simulink model "Chaine_de_conversion_eolienne_25kw"  (R2024a)
settings: Solver=FixedStepAuto  StartTime=0.0  StopTime=10  FixedStep=Ts  RelTol=1e-3
undefined symbols (not defined in the file): A1, A2, A3, A4, A5, A6, C_dc, f, F, G, J, J_PMSG, ki_id_grid, ki_iq_grid, ki_isd, ki_omega, ki_PLL, ki_Q, ki_vdc, kp_id_grid, kp_iq_grid, kp_isd, kp_omega, kp_PLL, kp_Q, kp_vdc, Kt, Lf, Ls, p, Phi_r, R, Rf, rho, Rs, S, Ts, Vdc_ref
libraries: eeGeneralControl x12, slpidlib x8, spsThreePhaseVIMeasurementLib x3, eeTransforms x3, spsCurrentMeasurementLib x3, spsVoltageMeasurementLib x3, spsUniversalBridgeLib x2, spsPWMGenerator2LevelLib x2, powerlib_extras x2, spsRMSLib x2, spsTHDLib x2, spsThreePhaseSeriesRLCBranchLib x1
(part 1 of 2)
settings Model: Creator=K Edd Edd  LastModifiedBy=K Edd Edd
settings DataIOCC: SignalLogging=off  DSMLogging=off  ReturnWorkspaceOutputs=off

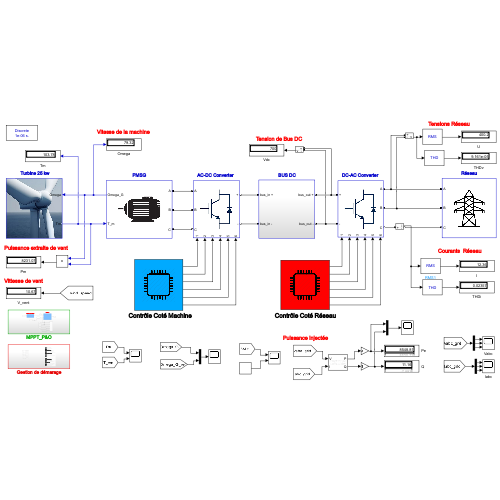
[thumbnail: Simulink's stored preview of the top-level diagram]
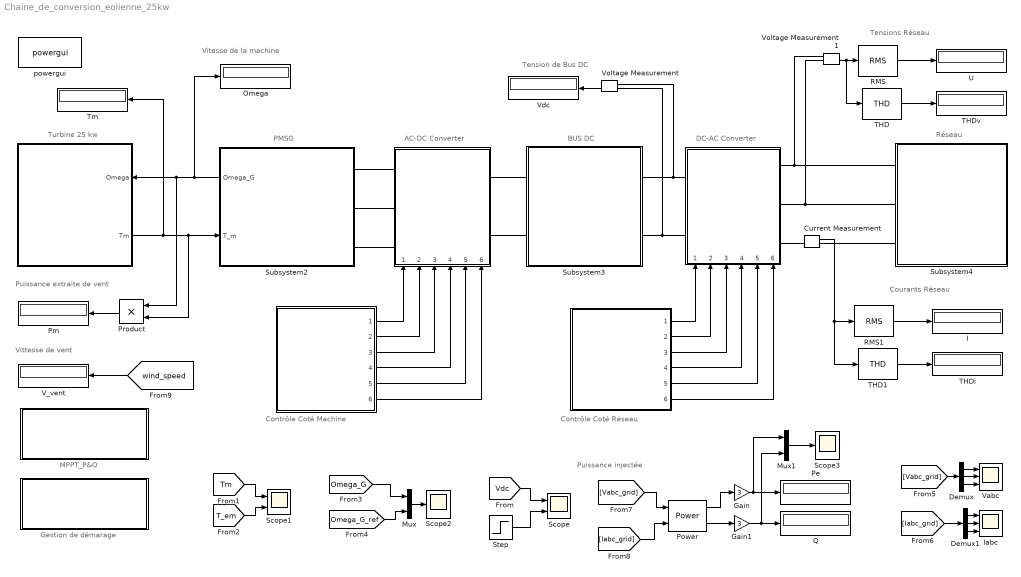
== system Chaine_de_conversion_eolienne_25kw ==
  note: Courants Réseau
  note: MPPT_P&O
  note: Turbine 25 kw
  note: PMSG
  note: AC-DC Converter
  note: BUS DC
  note: DC-AC Converter
  note: Réseau
  note: Gestion de démarage
  note: Contrôle Coté Machine
  note: Tensions Réseau
  note: Puissance injectée
  note: Tension de Bus DC
  note: Vitesse de la machine
  note: Puissance extraite de vent
  note: Contrôle Coté Réseau
  note: Vittesse de vent
  "  " : Subsystem
      settings: PortSchema="{\"entries\":[{\"content\":{\"sides\":[{\"content\":{\"connectorIds\":[\"LConn1\",\"LConn2\",\"LConn3\"]},\"type\":\"ConnectorPlacement.EquallySpacedRectSide\",\"uuid\":\"aa5a1e19-58e8-4f63-9a1b-77e9bc10e920\"},{\"content\":{\"connectorIds\":[\"RConn1\",\"RConn2\"],\"side\":\"RIGHT\"},\"type\":\"ConnectorPlacement.EquallySpacedRectSide\",\"uuid\":\"2d85d2be-ece1-4429-a3f7-d4ed68196552\"},{\"content\":{\"side\":\"TOP\"},\"type\":\"ConnectorPlacement.EquallySpacedRectSide\",\"uuid\":\"982ebd7b-1595-4ee8-b406-473be6344857\"},{\"content\":{\"connectorIds\":[\"In1\",\"In2\",\"In3\",\"In4\",\"In5\",\"In6\"],\"side\":\"BOTTOM\"},\"type\":\"ConnectorPlacement.EquallySpacedRectSide\",\"uuid\":\"f79fcda1-556e-4eeb-b27d-f3a2253a7ec4\"}]},\"type\":\"ConnectorPlacement.EquallySpacedConnector\",\"uuid\":\"743085b1-d620-4124-a445-722ff99a9231\"}],\"packageUris\":[\"http://schema.mathworks.com/mf0/Connector/R2020b\"],\"version\":\"1.0\"}"
      mask Display: image('Bridge_3ph.png', [0,0,0,0,90,90]);
  "   " : Subsystem
      settings: PortSchema="{\"entries\":[{\"content\":{\"sides\":[{\"content\":{},\"type\":\"ConnectorPlacement.EquallySpacedRectSide\",\"uuid\":\"46343f75-74e6-4f4c-9efc-4b43e6213925\"},{\"content\":{\"connectorIds\":[\"In1\",\"Out1\"],\"side\":\"RIGHT\"},\"type\":\"ConnectorPlacement.EquallySpacedRectSide\",\"uuid\":\"10880a8c-ba30-44f8-b93e-97455e8769b4\"},{\"content\":{\"side\":\"TOP\"},\"type\":\"ConnectorPlacement.EquallySpacedRectSide\",\"uuid\":\"fc9f6e01-6aae-438b-b3e4-23506a1fb9e3\"}]},\"type\":\"ConnectorPlacement.EquallySpacedConnector\",\"uuid\":\"29e446f6-be91-4db2-b818-9d2408c26281\"}],\"packageUris\":[\"http://schema.mathworks.com/mf0/Connector/R2020b\"],\"version\":\"1.0\"}"
      mask Display: image('Turbine.jpg');
  "    " : Subsystem
  "      " : Subsystem
  "         " : Subsystem
      settings: PortSchema="{\"entries\":[{\"content\":{\"sides\":[{\"content\":{\"connectorIds\":[\"LConn1\",\"LConn2\"]},\"type\":\"ConnectorPlacement.EquallySpacedRectSide\",\"uuid\":\"6a59fa23-55cb-493a-902b-27daa7c75780\"},{\"content\":{\"connectorIds\":[\"RConn1\",\"RConn2\",\"RConn3\"],\"side\":\"RIGHT\"},\"type\":\"ConnectorPlacement.EquallySpacedRectSide\",\"uuid\":\"f4ee7100-af9b-4531-bfab-eaffe06050e9\"},{\"content\":{\"side\":\"TOP\"},\"type\":\"ConnectorPlacement.EquallySpacedRectSide\",\"uuid\":\"b4ec731b-d05c-4ff1-948d-ff2fdeb075f1\"},{\"content\":{\"connectorIds\":[\"In1\",\"In2\",\"In3\",\"In4\",\"In5\",\"In6\"],\"side\":\"BOTTOM\"},\"type\":\"ConnectorPlacement.EquallySpacedRectSide\",\"uuid\":\"1fd09039-83e1-473e-9ccb-1d87c041e7c6\"}]},\"type\":\"ConnectorPlacement.EquallySpacedConnector\",\"uuid\":\"54ae46ec-08f8-45c2-a8da-c49a7efba60c\"}],\"packageUris\":[\"http://schema.mathworks.com/mf0/Connector/R2020b\"],\"version\":\"1.0\"}"
      mask Display: image('Bridge_3ph.png', [0,0,0,0,90,90]);
  "                 " : Subsystem
      settings: PortSchema="{\"entries\":[{\"content\":{\"sides\":[{\"content\":{},\"type\":\"ConnectorPlacement.EquallySpacedRectSide\",\"uuid\":\"68bdff09-e8ec-4d6d-b05e-55201ee357f5\"},{\"content\":{\"side\":\"RIGHT\"},\"type\":\"ConnectorPlacement.EquallySpacedRectSide\",\"uuid\":\"a14a2bca-9db8-408e-b5bf-8e3869a2fb13\"},{\"content\":{\"connectorIds\":[\"Out1\",\"Out2\",\"Out3\",\"Out4\",\"Out5\",\"Out6\"],\"side\":\"TOP\"},\"type\":\"ConnectorPlacement.EquallySpacedRectSide\",\"uuid\":\"600d12f1-b4e8-4864-955c-a539efb19c99\"}]},\"type\":\"ConnectorPlacement.EquallySpacedConnector\",\"uuid\":\"05b2b3d9-6bdc-4d72-9457-a6c68afa543f\"}],\"packageUris\":[\"http://schema.mathworks.com/mf0/Connector/R2020b\"],\"version\":\"1.0\"}"
      mask Display: image('Cotroller.jpg', [0,0,0,0,70,70]);
  "                       " : Subsystem
      settings: PortSchema="{\"entries\":[{\"content\":{\"sides\":[{\"content\":{},\"type\":\"ConnectorPlacement.EquallySpacedRectSide\",\"uuid\":\"68bdff09-e8ec-4d6d-b05e-55201ee357f5\"},{\"content\":{\"side\":\"RIGHT\"},\"type\":\"ConnectorPlacement.EquallySpacedRectSide\",\"uuid\":\"a14a2bca-9db8-408e-b5bf-8e3869a2fb13\"},{\"content\":{\"connectorIds\":[\"Out1\",\"Out2\",\"Out3\",\"Out4\",\"Out5\",\"Out6\"],\"side\":\"TOP\"},\"type\":\"ConnectorPlacement.EquallySpacedRectSide\",\"uuid\":\"600d12f1-b4e8-4864-955c-a539efb19c99\"}]},\"type\":\"ConnectorPlacement.EquallySpacedConnector\",\"uuid\":\"05b2b3d9-6bdc-4d72-9457-a6c68afa543f\"}],\"packageUris\":[\"http://schema.mathworks.com/mf0/Connector/R2020b\"],\"version\":\"1.0\"}"
      mask Display: image('Cotroller.jpg', [0,0,0,0,70,70]);
  Current Measurement : spsCurrentMeasurementLib/Current Measurement  PhasorSimulation=off  OutputType=Complex  PSBequivalent=0
  Demux : Demux  Outputs=3
  Demux1 : Demux  Outputs=3
  Gain : Gain  Gain=3
  Gain1 : Gain  Gain=3
  I : Display
  Iabc : Scope  NumInputPorts=3
  Mux : Mux  Inputs=2
  Mux1 : Mux  Inputs=2
  Omega : Display
  Pe : Display
      settings: Format=bank
  Pm : Display
      settings: Format=bank
  Power : spsPowerLib/Power  Freq=50  Vinit=[0, 0]  Iinit=[0, 0]  Ts=0
  Product : Product
  Q : Display
  RMS : spsRMSLib/RMS  TrueRMS=on  Freq=50  RMSInit=0  Ts=Ts
  RMS1 : spsRMSLib/RMS  TrueRMS=on  Freq=50  RMSInit=0  Ts=Ts
  Scope : Scope  NumInputPorts=2
  Scope1 : Scope  NumInputPorts=2
  Scope2 : Scope
  Scope3 : Scope
  Step : Step  Time=1e-8  Before=1e-8  After=700  SampleTime=0
  Subsystem2 : Subsystem
      settings: PortSchema="{\"entries\":[{\"content\":{\"sides\":[{\"content\":{\"connectorIds\":[\"Out1\",\"In1\"]},\"type\":\"ConnectorPlacement.EquallySpacedRectSide\",\"uuid\":\"3f25ae88-b85d-4aa8-83e0-c8881128a15f\"},{\"content\":{\"connectorIds\":[\"RConn1\",\"RConn2\",\"RConn3\"],\"side\":\"RIGHT\"},\"type\":\"ConnectorPlacement.EquallySpacedRectSide\",\"uuid\":\"21769176-b893-4bdb-b404-3c9a8a9ec7d7\"},{\"content\":{\"side\":\"TOP\"},\"type\":\"ConnectorPlacement.EquallySpacedRectSide\",\"uuid\":\"6b86daf7-1109-4b9d-a4e1-050e61d06be5\"}]},\"type\":\"ConnectorPlacement.EquallySpacedConnector\",\"uuid\":\"4237b530-1620-4b33-bc88-1364db079d0f\"}],\"packageUris\":[\"http://schema.mathworks.com/mf0/Connector/R2020b\"],\"version\":\"1.0\"}"
      mask Display: image('Machine.jpg');
  Subsystem3 : Subsystem
  Subsystem4 : Subsystem
      mask Display: image('Grid.jpg', [0,0,0,0,80,80]);
  THD : spsTHDLib/THD  Freq=50  Ts=0
  THD1 : spsTHDLib/THD  Freq=50  Ts=0
  THDi : Display
  THDv : Display
  Tm : Display
      settings: Format=bank
  U : Display
  V_vent : Display
      settings: Format=bank
  Vabc : Scope  NumInputPorts=3
  Vdc : Display
  Voltage Measurement : spsVoltageMeasurementLib/Voltage Measurement  PhasorSimulation=off  OutputType=Complex  PSBequivalent=0
  Voltage Measurement1 : spsVoltageMeasurementLib/Voltage Measurement  PhasorSimulation=off  OutputType=Complex  PSBequivalent=0
  powergui : sps_lib/powergui  Priority=1  SimulationMode=Discrete  SampleTime=Ts  frequency=60  Iterations=50  frequencyindice=0  Pbase=100e6  ErrMax=1e-4  UnitsV=kV  UnitsW=MW  buscounter=0  FunctionMessages=off  echomessages=off  EnableUseOfTLC=off  CurrentSourceSwitches=off  DisableSnubberDevices=off  DisableRonSwitches=off  DisableVfSwitches=off  DisplayEquations=off  AutomaticDiscreteSolvers=off  SolverType=Tustin/Backward Euler (TBE)  Interpol=off  ExternalGateDelay=off  methode=off  Ts=100  x0status=blocks  SPID=on  SwTol=0  HookPort=off  NonlinearTolerance=1e-4  nMaxIteration=100  ContinueOnMaxIteration=off  RestoreLinks=warning  ResistiveCurrentMeasurement=off  Frange=[0:2:500]  Ylog=off  Xlog=on  ShowGrid=off  save=off  variable=ZData  structure=0  ZoomFFT=off  StartTime=0.0  cycles=1  DisplayStyle=1  fundamental=60  FreqAxis=off  MaxFrequency=1000  frequencyindicesteady=1  RmsSteady=1  display=off
  wires:
  "                 "/1(" ") -> "  "/1(Input)
  "                 "/2("  ") -> "  "/2(Input1)
  "                 "/3("   ") -> "  "/3(Input2)
  "                 "/4("    ") -> "  "/4(Input3)
  "                 "/5("     ") -> "  "/5(Input4)
  "                 "/6("       ") -> "  "/6(Input5)
  "   "/1(Tm) -> Tm/1, Product/2, Subsystem2/1(T_m)
  "                       "/4("    ") -> "         "/4(Input3)
  "                       "/6("      ") -> "         "/6(Input5)
  "                       "/3("   ") -> "         "/3(Input2)
  "                       "/1(" ") -> "         "/1(Input)
  "                       "/2("  ") -> "         "/2(Input1)
  "                       "/5("     ") -> "         "/5(Input4)
  Voltage Measurement/1 -> Vdc/1
  Voltage Measurement1/1 -> RMS/1, THD/1
  RMS/1 -> U/1
  THD/1 -> THDv/1
  Demux1/3 -> Iabc/3
  Demux/1 -> Vabc/1
  [Iabc_grid] -> Demux1/1
  Demux1/2 -> Iabc/2
  Demux/3 -> Vabc/3
  Demux1/1 -> Iabc/1
  Demux/2 -> Vabc/2
  [Vabc_grid] -> Demux/1
  [Vdc] -> Scope/1
  Step/1 -> Scope/2
  [T_em] -> Scope1/2
  [Tm] -> Scope1/1
  Product/1 -> Pm/1
  Subsystem2/1(Omega_G) -> "   "/1(Omega), Product/1, Omega/1
  [Vabc_grid] -> Power/1
  [Iabc_grid] -> Power/2
  Power/1 -> Gain/1
  Power/2 -> Gain1/1
  Gain1/1 -> Mux1/2, Q/1
  THD1/1 -> THDi/1
  RMS1/1 -> I/1
  Current Measurement/1 -> RMS1/1, THD1/1
  [wind_speed] -> V_vent/1
  [Omega_G] -> Mux/1
  Mux/1 -> Scope2/1
  [Omega_G_ref] -> Mux/2
  Mux1/1 -> Scope3/1
  Gain/1 -> Mux1/1, Pe/1
  connections:
  Subsystem2/RConn1 -- "  "/LConn1
  Subsystem2/RConn2 -- "  "/LConn2
  Subsystem2/RConn3 -- "  "/LConn3
  Subsystem3/LConn1 -- "  "/RConn1
  "  "/RConn2 -- Subsystem3/LConn2
  "         "/LConn1 -- Voltage Measurement/LConn1 -- Subsystem3/RConn1
  "         "/LConn2 -- Voltage Measurement/LConn2 -- Subsystem3/RConn2
  Subsystem4/LConn1 -- Voltage Measurement1/LConn1 -- "         "/RConn1
  Subsystem4/LConn2 -- Voltage Measurement1/LConn2 -- "         "/RConn2
  Current Measurement/LConn1 -- "         "/RConn3
  Current Measurement/RConn1 -- Subsystem4/LConn3

== system Chaine_de_conversion_eolienne_25kw/   ==
  note: Redresseur actif
  note: Bus DC
  note: Tensions Machine
  Input : Inport
  Input1 : Inport  Port=2
  Input2 : Inport  Port=3
  Input3 : Inport  Port=4
  Input4 : Inport  Port=5
  Input5 : Inport  Port=6
  "  " : spsUniversalBridgeLib/Universal Bridge  Arms=3  SnubberResistance=1e7  SnubberCapacitance=inf  Device=IGBT / Diodes  Ron=1e-2  Lon=0  ForwardVoltages="[  0  0  ]"  ForwardVoltage=0  GTOparameters=[ 10e-6 , 20e-6 ]  IGBTparameters=[ 0 , 0 ]  Measurements=None  Measurements_2=None  converterType=Rectifier
  Mux : Mux  Inputs=6
  A : PMIOPort  Side=Left
  B : PMIOPort  Port=2  Side=Left
  C : PMIOPort  Port=3  Side=Left
  + : PMIOPort  Port=4  Side=Right
  - : PMIOPort  Port=5  Side=Right
  wires:
  Input/1 -> Mux/1
  Input1/1 -> Mux/2
  Input2/1 -> Mux/3
  Input3/1 -> Mux/4
  Input4/1 -> Mux/5
  Input5/1 -> Mux/6
  Mux/1 -> "  "/1
  connections:
  -/RConn1 -- "  "/RConn2
  B/RConn1 -- "  "/LConn2
  A/RConn1 -- "  "/LConn1
  C/RConn1 -- "  "/LConn3
  +/RConn1 -- "  "/RConn1

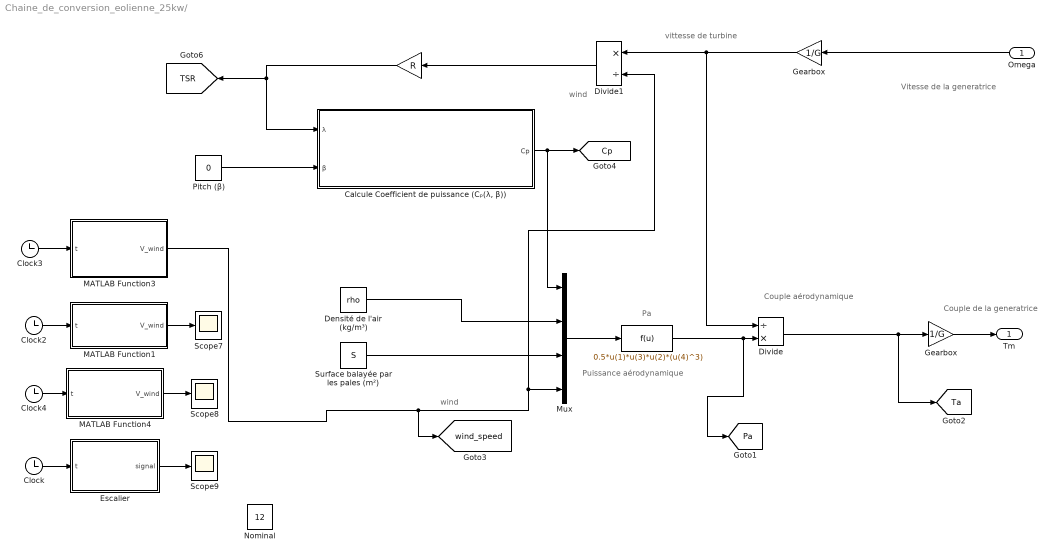
== system Chaine_de_conversion_eolienne_25kw/    ==
  note: Couple de la generatrice
  note: Puissance aérodynamique
  note: wind
  note: vittesse de turbine
  note: Couple aérodynamique
  note: Vitesse de la generatrice
  note: Pa
  note: wind
  Omega : Inport
  "  " : Fcn  Expr=0.5*u(1)*u(3)*u(2)*(u(4)^3)
  "   " : Gain  Gain=R
  "Calcule Coefficient de puissance (Cₚ(λ, β))" : Subsystem
  Clock{,2..4} (4 alike) : Clock
  Densité de l'air (kg/m³) : Constant  Value=rho
  Divide : Product  Inputs=/*
  Divide1 : Product  Inputs=*/
  Escalier : MATLAB Function  TreatAsAtomicUnit=on
  Gearbox : Gain  Gain=1/G
  "Gearbox   " : Gain  Gain=1/G
  MATLAB Function1 : MATLAB Function  TreatAsAtomicUnit=on  SystemSampleTime=0.001
  MATLAB Function3 : MATLAB Function  TreatAsAtomicUnit=on  SystemSampleTime=0.001
  MATLAB Function4 : MATLAB Function  TreatAsAtomicUnit=on  SystemSampleTime=0.001
  Mux : Mux
  Nominal : Constant  Value=12
  "Pitch (β) " : Constant  Value=0
  Scope7 : Scope
  Scope8 : Scope
  Scope9 : Scope
  Surface balayée par les pales (m²) : Constant  Value=S
  Tm : Outport
  tag scope: Cp=global, Pa=global, TSR=global, Ta=global, wind_speed=global
  wires:
  Clock2/1 -> MATLAB Function1/1(t)
  Clock3/1 -> MATLAB Function3/1(t)
  Clock4/1 -> MATLAB Function4/1(t)
  Surface balayée par les pales (m²)/1 -> Mux/3
  "Calcule Coefficient de puissance (Cₚ(λ, β))"/1(Cp) -> Mux/1, [Cp]
  MATLAB Function3/1(V_wind) -> Divide1/2, Mux/4, [wind_speed]
  Divide/1 -> [Ta], "Gearbox   "/1
  "Pitch (β) "/1 -> "Calcule Coefficient de puissance (Cₚ(λ, β))"/2(β)
  Gearbox/1 -> Divide/1, Divide1/1
  Densité de l'air (kg/m³)/1 -> Mux/2
  "   "/1 -> [TSR], "Calcule Coefficient de puissance (Cₚ(λ, β))"/1(λ)
  "Gearbox   "/1 -> Tm/1
  Divide1/1 -> "   "/1
  Mux/1 -> "  "/1
  "  "/1 -> [Pa], Divide/2
  Omega/1 -> Gearbox/1
  Clock/1 -> Escalier/1(t)
  MATLAB Function1/1(V_wind) -> Scope7/1
  MATLAB Function4/1(V_wind) -> Scope8/1
  Escalier/1(signal) -> Scope9/1

== system Chaine_de_conversion_eolienne_25kw/     ==
  note: 1. Cmd_Breaker_Grid (Disjoncteur Réseau)
      | Type : Physique (Bloc Three-Phase Breaker ).
      | Rôle : Connecte physiquement le filtre RL au réseau.
      | État 0 : Ouvert (Système isolé).
      | État 1 : Fermé (Système couplé).
      | 2. Enable_PWM_GSC (Activation Onduleur Réseau)
      | Type : Logique (Port Enable du générateur PWM ou des IGBTs).
      | Rôle : Autorise l'envoi des impulsions aux gâchettes côté réseau.
      | État 0 : Bloqué (Les IGBTs sont ouverts, l'onduleur agit comme un pont de diodes passif).
      | État 1 : Actif (L'onduleur module la tension).
      | 3. Mode_Injection_GSC (Sélecteur de Référence Courant)
      | Type : Logique (Bloc Switch dans la commande).
      | Rôle : Bascule entre le mode "Synchronisation" (Courant nul) et le mode "Régulation Bus DC".
      | État 0 : Force
      | Id_ref=0 I d _ ref ​ =0 et
      | Iq_ref=0 I q _ ref ​ =0
      | .
      | État 1ser : Connecte la sortie du PI
      | Vdc V dc ​ à l'entrée
      | Id_ref I d _ ref ​ (Démarrage de l'injection).
      | 4. Enable_PWM_MSC (Activation Redresseur Machine)
      | Type : Logique (Port Enable du PWM côté machine).
      | Rôle : Autorise le contrôle de la génératrice PMSG.
      | État 0 : Bloqué (Roue libre, pas de couple électromagnétique).
      | État 1 : Actif (La machine est contrôlée).
      | 5. Enable_MPPT (Activation de la charge)
      | Type : Logique (Celui que nous avons créé pour votre fonction MPPT).
      | Rôle : Autorise la prise de couple (Feed-Forward et algo P&O).
      | État 0 : Référence Vitesse =
      | ΩmesΩ mes ​ (couple nul).
      | État 1 : Référence Vitesse = MPPT (couple actif).
  Constant{,1..3} (4 alike) : Constant
  Constant4 : Constant  Value=0
  tag scope: Cmd_Breaker_Grid=global, Enable_MPPT=global, Enable_PWM_GSC=global, Enable_PWM_MSC=global, Mode_Injection_GSC=global
  wires:
  Constant/1 -> [Cmd_Breaker_Grid]
  Constant1/1 -> [Enable_PWM_GSC]
  Constant2/1 -> [Mode_Injection_GSC]
  Constant3/1 -> [Enable_PWM_MSC]
  Constant4/1 -> [Enable_MPPT]

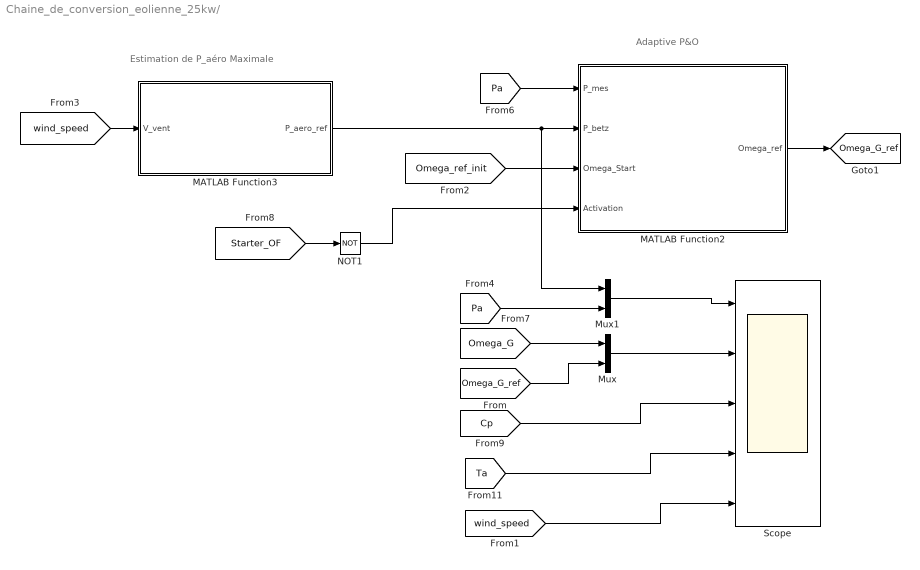
== system Chaine_de_conversion_eolienne_25kw/       ==
  note: Estimation de P_aéro Maximale
  note: Adaptive P&O
  MATLAB Function2 : MATLAB Function  TreatAsAtomicUnit=on  SystemSampleTime=0.001
  MATLAB Function3 : MATLAB Function  TreatAsAtomicUnit=on  SystemSampleTime=0.001
  Mux : Mux  Inputs=2
  Mux1 : Mux  Inputs=2
  NOT1 : Logic  Operator=NOT  IconShape=distinctive  AllPortsSameDT=off  OutDataTypeStr=boolean
  Scope : Scope  NumInputPorts=5
  tag scope: Omega_G_ref=global
  wires:
  [Pa] -> MATLAB Function2/1(P_mes)
  MATLAB Function2/1(Omega_ref) -> [Omega_G_ref]
  MATLAB Function3/1(P_aero_ref) -> Mux1/1, MATLAB Function2/2(P_betz)
  [wind_speed] -> MATLAB Function3/1(V_vent)
  [Pa] -> Mux1/2
  [Omega_G_ref] -> Mux/2
  [Omega_G] -> Mux/1
  Mux1/1 -> Scope/1
  Mux/1 -> Scope/2
  [Starter_OF] -> NOT1/1
  [Cp] -> Scope/3
  [Ta] -> Scope/4
  [wind_speed] -> Scope/5
  [Omega_ref_init] -> MATLAB Function2/3(Omega_Start)
  NOT1/1 -> MATLAB Function2/4(Activation)

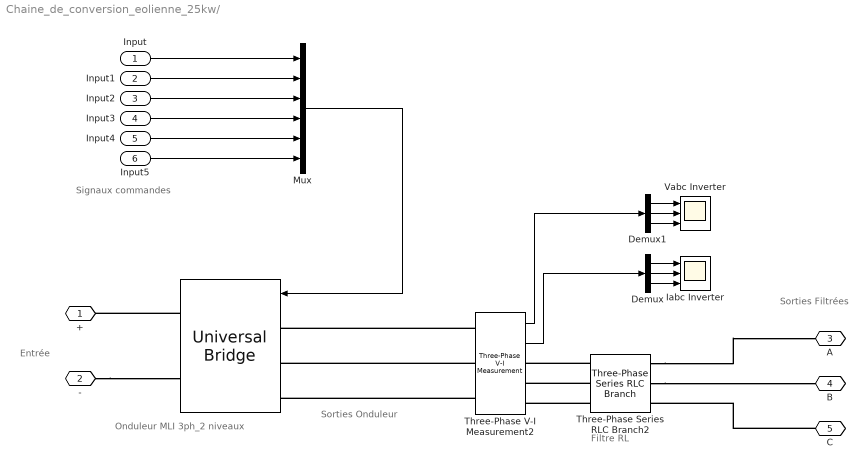
== system Chaine_de_conversion_eolienne_25kw/          ==
  note: Signaux commandes
  note: Entrée
  note: Sorties Filtrées
  note: Sorties Onduleur
  note: Onduleur MLI 3ph_2 niveaux
  note: Filtre RL
  Input : Inport
  Input1 : Inport  Port=2
  Input2 : Inport  Port=3
  Input3 : Inport  Port=4
  Input4 : Inport  Port=5
  Input5 : Inport  Port=6
  "    " : spsUniversalBridgeLib/Universal Bridge  Arms=3  SnubberResistance=1e7  SnubberCapacitance=inf  Device=IGBT / Diodes  Ron=1e-2  Lon=0  ForwardVoltages="[  0  0  ]"  ForwardVoltage=0  GTOparameters=[ 10e-6 , 20e-6 ]  IGBTparameters=[ 0 , 0 ]  Measurements=None  Measurements_2=None  converterType=Rectifier
  Demux : Demux  Outputs=3
  Demux1 : Demux  Outputs=3
  Iabc Inverter : Scope  NumInputPorts=3
  Mux : Mux  Inputs=6
  Three-Phase Series RLC Branch2 : spsThreePhaseSeriesRLCBranchLib/Three-Phase Series RLC Branch  LConnTagsString=A|B|C  RConnTagsString=A|B|C  BranchType=RL  Resistance=Rf  Inductance=Lf  Capacitance=1e-6  Measurements=None
  Three-Phase V-I Measurement2 : spsThreePhaseVIMeasurementLib/Three-Phase V-I Measurement  VoltageMeasurement=phase-to-ground  SetLabelV=off  LabelV=Vabc_Inverter  Vpu=off  VpuLL=off  CurrentMeasurement=yes  SetLabelI=off  LabelI=Iabc_Inverter  Ipu=off  Pbase=100e6  Vbase=500e3  OutputType=Complex  PhasorSimulation=off  PSBequivalent=0
  Vabc Inverter : Scope  NumInputPorts=3
  + : PMIOPort  Side=Left
  - : PMIOPort  Port=2  Side=Left
  A : PMIOPort  Port=3  Side=Right
  B : PMIOPort  Port=4  Side=Right
  C : PMIOPort  Port=5  Side=Right
  wires:
  Mux/1 -> "    "/1
  Input5/1 -> Mux/6
  Input4/1 -> Mux/5
  Input3/1 -> Mux/4
  Input2/1 -> Mux/3
  Input1/1 -> Mux/2
  Input/1 -> Mux/1
  Three-Phase V-I Measurement2/2 -> Demux/1
  Demux/2 -> Iabc Inverter/2
  Demux/1 -> Iabc Inverter/1
  Demux/3 -> Iabc Inverter/3
  Demux1/3 -> Vabc Inverter/3
  Demux1/1 -> Vabc Inverter/1
  Demux1/2 -> Vabc Inverter/2
  Three-Phase V-I Measurement2/1 -> Demux1/1
  connections:
  "    "/RConn1 -- +/RConn1
  -/RConn1 -- "    "/RConn2
  Three-Phase V-I Measurement2/LConn3 -- "    "/LConn3
  Three-Phase V-I Measurement2/LConn2 -- "    "/LConn2
  Three-Phase V-I Measurement2/LConn1 -- "    "/LConn1
  Three-Phase Series RLC Branch2/LConn1 -- Three-Phase V-I Measurement2/RConn1
  Three-Phase Series RLC Branch2/LConn2 -- Three-Phase V-I Measurement2/RConn2
  Three-Phase Series RLC Branch2/LConn3 -- Three-Phase V-I Measurement2/RConn3
  Three-Phase Series RLC Branch2/RConn1 -- A/RConn1
  Three-Phase Series RLC Branch2/RConn2 -- B/RConn1
  C/RConn1 -- Three-Phase Series RLC Branch2/RConn3

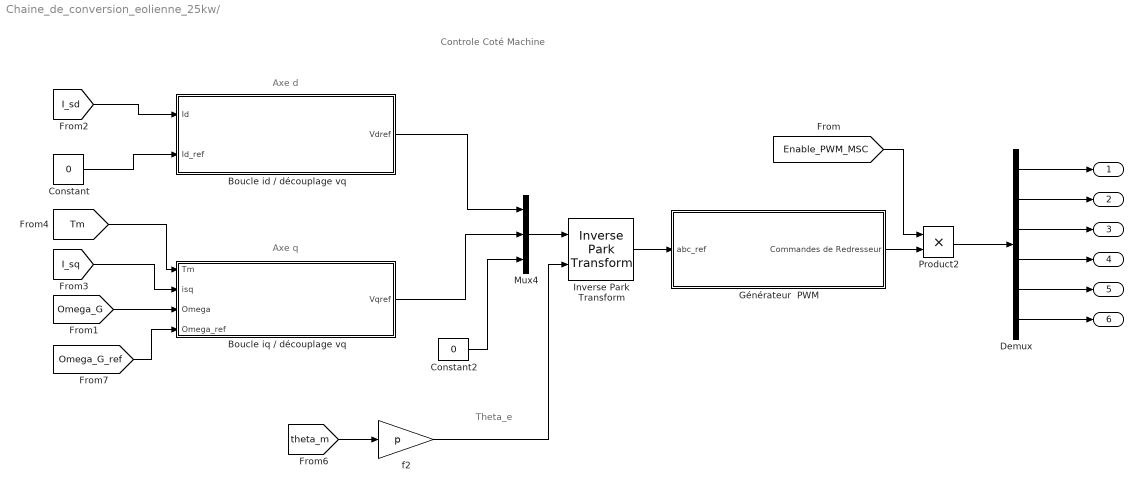
== system Chaine_de_conversion_eolienne_25kw/                  ==
  note: Axe q
  note: Axe d
  note: Theta_e
  note: Controle Coté Machine
  Boucle id / découplage vq : Subsystem
  Boucle iq / découplage vq : Subsystem
  Constant : Constant  Value=0
  Constant2 : Constant  Value=0
  Demux : Demux  Outputs=6
  Générateur  PWM : Subsystem
  Inverse Park Transform : eeTransforms/Inverse Park Transform  AxisAlignment=Q-axis  PowerInvariant=off
      settings: LibrarySourceBlock=|
      | ee_sl_lib/Mathematical
      | Transforms/Inverse
      | Park Transform
  Mux4 : Mux  Inputs=3
  Product2 : Product
  f2 : Gain  Gain=p  SaturateOnIntegerOverflow=on  OutDataTypeStr=Inherit: Same as input  ParamDataTypeStr=Inherit: Same as input
  " " : Outport
  "  " : Outport  Port=2
  "   " : Outport  Port=3
  "    " : Outport  Port=4
  "     " : Outport  Port=5
  "       " : Outport  Port=6
  wires:
  Constant2/1 -> Mux4/3
  Inverse Park Transform/1 -> Générateur  PWM/1(abc_ref)
  [theta_m] -> f2/1
  [I_sd] -> Boucle id / découplage vq/1(Id)
  [I_sq] -> Boucle iq / découplage vq/2(isq)
  [Omega_G_ref] -> Boucle iq / découplage vq/4(Omega_ref)
  [Omega_G] -> Boucle iq / découplage vq/3(Omega)
  Boucle id / découplage vq/1(Vdref) -> Mux4/1
  Boucle iq / découplage vq/1(Vqref) -> Mux4/2
  Product2/1 -> Demux/1
  f2/1 -> Inverse Park Transform/2
  Demux/1 -> " "/1
  Demux/2 -> "  "/1
  Demux/3 -> "   "/1
  Demux/4 -> "    "/1
  Demux/5 -> "     "/1
  Demux/6 -> "       "/1
  Mux4/1 -> Inverse Park Transform/1
  Générateur  PWM/1(Commandes de Redresseur) -> Product2/2
  [Enable_PWM_MSC] -> Product2/1
  Constant/1 -> Boucle id / découplage vq/2(Id_ref)
  [Tm] -> Boucle iq / découplage vq/1(Tm)

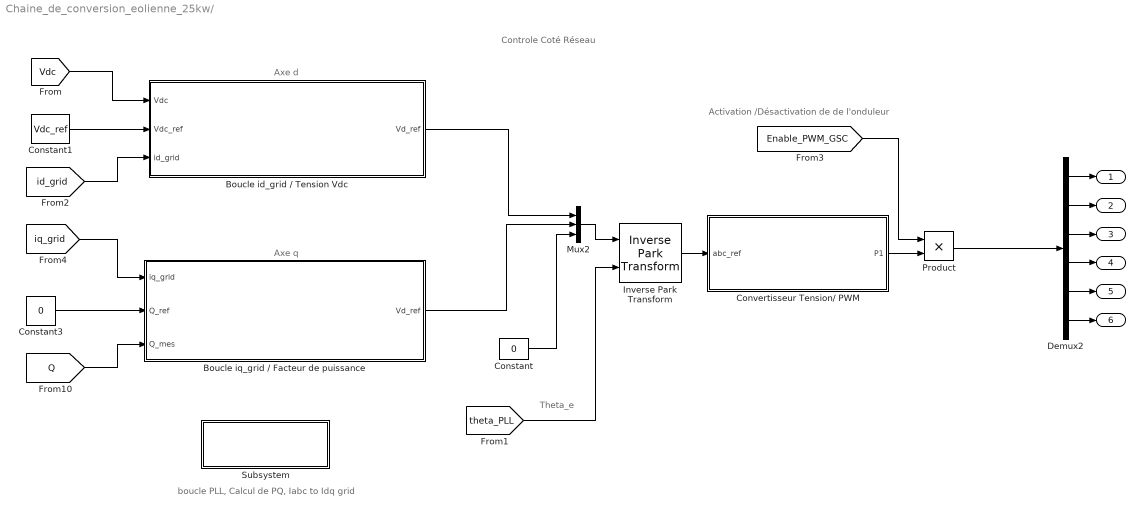
== system Chaine_de_conversion_eolienne_25kw/                        ==
  note: Controle Coté Réseau
  note: Activation /Désactivation de de l'onduleur
  note: Axe d
  note: boucle PLL, Calcul de PQ, Iabc to Idq grid
  note: Axe q
  note: Theta_e
  Boucle id_grid / Tension Vdc : Subsystem
  Boucle iq_grid / Facteur de puissance : Subsystem
  Constant : Constant  Value=0
  Constant1 : Constant  Value=Vdc_ref
  Constant3 : Constant  Value=0
  "Convertisseur Tension/ PWM " : Subsystem
  Demux2 : Demux  Outputs=6
  Inverse Park Transform : eeTransforms/Inverse Park Transform  AxisAlignment=Q-axis  PowerInvariant=off
      settings: LibrarySourceBlock=|
      | ee_sl_lib/Mathematical
      | Transforms/Inverse
      | Park Transform
  Mux2 : Mux  Inputs=3
  Product : Product
  Subsystem : Subsystem
  " " : Outport
  "  " : Outport  Port=2
  "   " : Outport  Port=3
  "    " : Outport  Port=4
  "     " : Outport  Port=5
  "      " : Outport  Port=6
  wires:
  [theta_PLL] -> Inverse Park Transform/2
  Mux2/1 -> Inverse Park Transform/1
  Constant/1 -> Mux2/3
  [id_grid] -> Boucle id_grid / Tension Vdc/3(id_grid)
  Constant1/1 -> Boucle id_grid / Tension Vdc/2(Vdc_ref)
  Constant3/1 -> Boucle iq_grid / Facteur de puissance/2(Q_ref)
  Inverse Park Transform/1 -> "Convertisseur Tension/ PWM "/1(abc_ref)
  Boucle iq_grid / Facteur de puissance/1(Vd_ref) -> Mux2/2
  Boucle id_grid / Tension Vdc/1(Vd_ref) -> Mux2/1
  Demux2/6 -> "      "/1
  Product/1 -> Demux2/1
  Demux2/3 -> "   "/1
  Demux2/5 -> "     "/1
  Demux2/1 -> " "/1
  Demux2/4 -> "    "/1
  Demux2/2 -> "  "/1
  [Vdc] -> Boucle id_grid / Tension Vdc/1(Vdc)
  [iq_grid] -> Boucle iq_grid / Facteur de puissance/1(iq_grid)
  [Q] -> Boucle iq_grid / Facteur de puissance/3(Q_mes)
  "Convertisseur Tension/ PWM "/1(P1) -> Product/2
  [Enable_PWM_GSC] -> Product/1

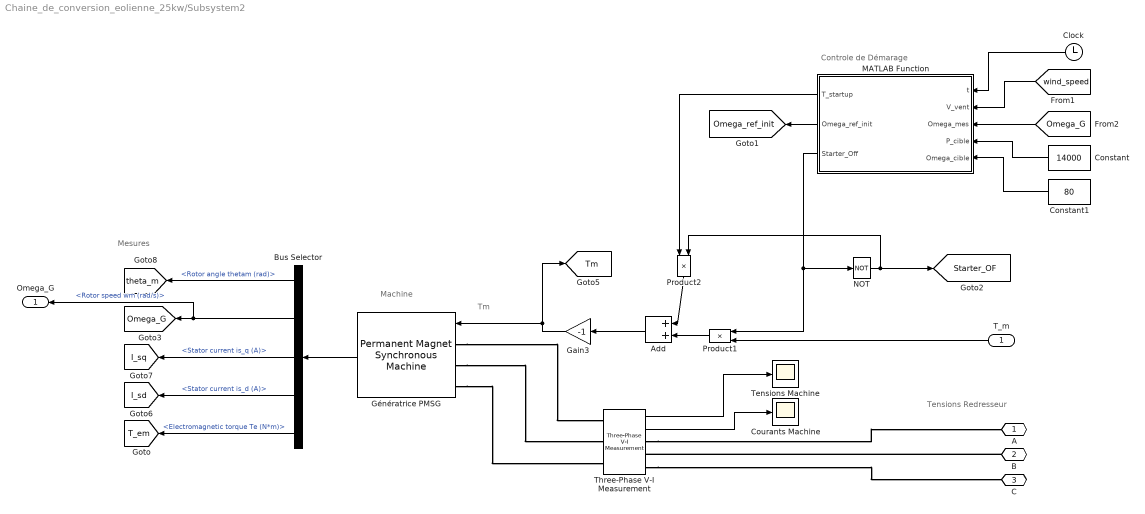
== system Chaine_de_conversion_eolienne_25kw/Subsystem2 ==
  note: Controle de Démarage
  note: Machine
  note: Tm
  note: Mesures
  note: Tensions Redresseur
  T_m : Inport
  Add : Sum
  Bus Selector : BusSelector  OutputSignals=Rotor angle thetam (rad),Rotor speed wm (rad/s),Stator current is_q (A),Stator current is_d (A),Electromagnetic torque Te (N*m)
  Clock : Clock
  Constant : Constant  Value=14000
  Constant1 : Constant  Value=80
  "Courants Machine " : Scope
  Gain3 : Gain  Gain=-1
  Génératrice PMSG : spsPermanentMagnetSynchronousMachineLib/Permanent Magnet Synchronous Machine  NbPhases=3  FluxDistribution=Sinusoidal  RotorType=Round  MechanicalLoad=Torque Tm  PresetModel=No  ShowDetailedParameters=on  MeasurementBus=off  Resistance=Rs  Inductance=8.5e-3  dqInductances=[8.5e-3,8.5e-3]  La=Ls  MachineConstant=Flux linkage established by magnets (V.s)  Flux=Phi_r  VoltageCst=86.6271  TorqueCst=0.7164  Flat=120  Mechanical=[J F p 0]  PolePairs=4  InitialConditions=[0.01 ,0, 0,0]  InitialConditions5ph=[0 0 0 0 0 0]  RefAngle=90 degrees behind phase A axis (modified Park)  IterativeDiscreteModel=Trapezoidal non iterative  TsBlock=-1  TsPowergui=0
  MATLAB Function : MATLAB Function  TreatAsAtomicUnit=on  SystemSampleTime=Ts
  NOT : Logic  Operator=NOT  IconShape=distinctive  AllPortsSameDT=off  OutDataTypeStr=boolean
  Product1 : Product
  Product2 : Product
  "Tensions Machine " : Scope
  Three-Phase V-I Measurement : spsThreePhaseVIMeasurementLib/Three-Phase V-I Measurement  VoltageMeasurement=phase-to-ground  SetLabelV=off  LabelV=Vabc  Vpu=off  VpuLL=off  CurrentMeasurement=yes  SetLabelI=off  LabelI=Iabc  Ipu=off  Pbase=100e6  Vbase=500e3  OutputType=Complex  PhasorSimulation=off  PSBequivalent=0
  A : PMIOPort  Side=Right
  B : PMIOPort  Port=2  Side=Right
  C : PMIOPort  Port=3  Side=Right
  Omega_G : Outport
  tag scope: I_sd=global, I_sq=global, Omega_G=global, Omega_ref_init=global, Starter_OF=global, T_em=global, Tm=global, theta_m=global
  wires:
  Bus Selector/1 -> [theta_m]  "<Rotor angle thetam (rad)>"
  Bus Selector/2 -> Omega_G/1, [Omega_G]  "<Rotor speed wm (rad/s)>"
  Génératrice PMSG/1 -> Bus Selector/1
  Bus Selector/4 -> [I_sd]  "<Stator current is_d (A)>"
  Bus Selector/5 -> [T_em]  "<Electromagnetic torque Te (N*m)>"
  Bus Selector/3 -> [I_sq]  "<Stator current is_q (A)>"
  Gain3/1 -> [Tm], Génératrice PMSG/1
  Three-Phase V-I Measurement/1 -> "Tensions Machine "/1
  Three-Phase V-I Measurement/2 -> "Courants Machine "/1
  Product1/1 -> Add/2
  MATLAB Function/3(Starter_Off) -> NOT/1, Product1/1
  MATLAB Function/2(Omega_ref_init) -> [Omega_ref_init]
  MATLAB Function/1(T_startup) -> Product2/1
  [Omega_G] -> MATLAB Function/3(Omega_mes)
  NOT/1 -> Product2/2, [Starter_OF]
  [wind_speed] -> MATLAB Function/2(V_vent)
  Product2/1 -> Add/1
  T_m/1 -> Product1/2
  Constant/1 -> MATLAB Function/4(P_cible)
  Constant1/1 -> MATLAB Function/5(Omega_cible)
  Add/1 -> Gain3/1
  Clock/1 -> MATLAB Function/1(t)
  connections:
  Génératrice PMSG/LConn1 -- Three-Phase V-I Measurement/LConn1
  Génératrice PMSG/LConn2 -- Three-Phase V-I Measurement/LConn2
  Génératrice PMSG/LConn3 -- Three-Phase V-I Measurement/LConn3
  Three-Phase V-I Measurement/RConn1 -- A/RConn1
  B/RConn1 -- Three-Phase V-I Measurement/RConn2
  Three-Phase V-I Measurement/RConn3 -- C/RConn1

== system Chaine_de_conversion_eolienne_25kw/Subsystem3 ==
  note: Filtre Redresseur
  C_dc : spsSeriesRLCBranchLib/Series RLC Branch  LConnTagsString=__new0  RConnTagsString=__new0  BranchType=C  Resistance=10  Inductance=1e-3  SetiL0=off  InitialCurrent=0  Capacitance=C_dc  Setx0=on  InitialVoltage=Vdc_ref  Measurements=None
  Current Measurement1 : spsCurrentMeasurementLib/Current Measurement  PhasorSimulation=off  OutputType=Complex  PSBequivalent=0
  Current Measurement2 : spsCurrentMeasurementLib/Current Measurement  PhasorSimulation=off  OutputType=Complex  PSBequivalent=0
  Voltage Measurement : spsVoltageMeasurementLib/Voltage Measurement  PhasorSimulation=off  OutputType=Complex  PSBequivalent=0
  bus_in + : PMIOPort  Side=Left
  bus_in - : PMIOPort  Port=2  Side=Left
  bus_out + : PMIOPort  Port=3  Side=Right
  bus_out - : PMIOPort  Port=4  Side=Right
  tag scope: I_ch=global, I_load_dc=global, Vdc=global
  wires:
  Voltage Measurement/1 -> [Vdc]
  Current Measurement2/1 -> [I_ch]
  Current Measurement1/1 -> [I_load_dc]
  connections:
  C_dc/LConn1 -- Current Measurement1/RConn1 -- Current Measurement2/LConn1
  C_dc/RConn1 -- bus_in -/RConn1 -- bus_out -/RConn1 -- Voltage Measurement/LConn2
  Current Measurement1/LConn1 -- bus_in +/RConn1
  Voltage Measurement/LConn1 -- Current Measurement2/RConn1 -- bus_out +/RConn1

== system Chaine_de_conversion_eolienne_25kw/Subsystem4 ==
  note: Disjoncteur Réseau
  note: Réseau
  Three-Phase V-I Measurement1 : spsThreePhaseVIMeasurementLib/Three-Phase V-I Measurement  VoltageMeasurement=phase-to-ground  SetLabelV=on  LabelV=Vabc_grid  Vpu=off  VpuLL=off  CurrentMeasurement=yes  SetLabelI=on  LabelI=Iabc_grid  Ipu=off  Pbase=100e6  Vbase=500e3  OutputType=Complex  PhasorSimulation=off  PSBequivalent=0
  Three-Phase Breaker : spsThreePhaseBreakerLib/Three-Phase Breaker  InitialState=open  SwitchA=on  SwitchB=on  SwitchC=on  SwitchTimes="[1/60  5/60]"  External=on  BreakerResistance=0.01  SnubberResistance=1e6  SnubberCapacitance=inf  Measurements=None
  Three-Phase Source : spsThreePhaseSourceLib/Three-Phase Source  InternalConnection=Yg  VoltagePhases=off  Voltage=400  PhaseAngle=0  Voltage_phases=[25e3 25e3 25e3]/sqrt(3)  PhaseAngles_phases=[0 -120 +120]  Frequency=50  NonIdealSource=on  SpecifyImpedance=off  Resistance=0.00000001  Inductance=0.00000001  ShortCircuitLevel=100e6  BaseVoltage=400  XRratio=7  BusType=swing  Pref=10e3  Qref=0  Prefabc=[10e3, 10e3, 10e3]  Qrefabc=[0, 0, 0]  Qmin=-inf  Qmax=inf
  A : PMIOPort  Side=Left
  B : PMIOPort  Port=2  Side=Left
  C : PMIOPort  Port=3  Side=Left
  wires:
  [Cmd_Breaker_Grid] -> Three-Phase Breaker/1
  connections:
  Three-Phase Breaker/RConn3 -- Three-Phase V-I Measurement1/LConn3
  Three-Phase V-I Measurement1/LConn2 -- Three-Phase Breaker/RConn2
  Three-Phase V-I Measurement1/LConn1 -- Three-Phase Breaker/RConn1
  B/RConn1 -- Three-Phase Breaker/LConn2
  C/RConn1 -- Three-Phase Breaker/LConn3
  A/RConn1 -- Three-Phase Breaker/LConn1
  Three-Phase Source/RConn1 -- Three-Phase V-I Measurement1/RConn1
  Three-Phase Source/RConn2 -- Three-Phase V-I Measurement1/RConn2
  Three-Phase Source/RConn3 -- Three-Phase V-I Measurement1/RConn3

== system Chaine_de_conversion_eolienne_25kw/   /Calcule Coefficient de puissance (Cₚ(λ, β)) ==
  λ : Inport
  β : Inport  Port=2
  " Cp(λ,β)" : Fcn  Expr=A1 * ( ((A2 * u(2)) - (A3 * u(1)) - A4) * exp(A5 * u(2)) + (A6 * u(3)) )
  1/λi : Fcn  Expr=(1 / (u(2) + (0.08 * u(1)))) - (0.035 / ((u(1)^3) + 1))
  Mux : Mux  Inputs=2
  Mux1 : Mux  Inputs=3
  Cp : Outport
  wires:
  Mux1/1 -> " Cp(λ,β)"/1
  Mux/1 -> 1/λi/1
  λ/1 -> Mux/2, Mux1/3
  β/1 -> Mux/1, Mux1/1
  1/λi/1 -> Mux1/2
  " Cp(λ,β)"/1 -> Cp/1

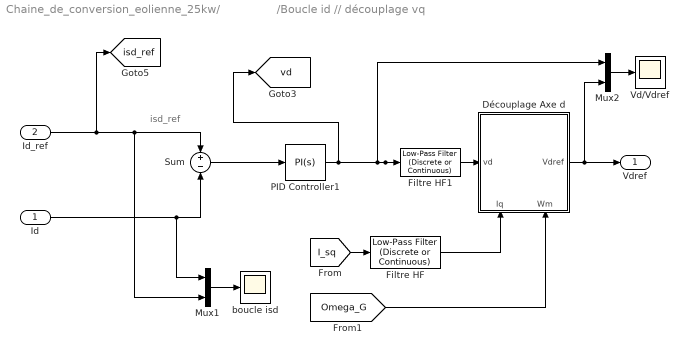
== system Chaine_de_conversion_eolienne_25kw/                 /Boucle id // découplage vq ==
  note: isd_ref
  Id : Inport
  Id_ref : Inport  Port=2
  " Vd/Vdref" : Scope
  Découplage Axe d : Subsystem
      settings: PortSchema="{\"entries\":[{\"content\":{\"sides\":[{\"content\":{\"connectorIds\":[\"In1\"]},\"type\":\"ConnectorPlacement.EquallySpacedRectSide\",\"uuid\":\"a35b541f-6c91-4579-89f1-6689e9beed7f\"},{\"content\":{\"connectorIds\":[\"Out1\"],\"side\":\"RIGHT\"},\"type\":\"ConnectorPlacement.EquallySpacedRectSide\",\"uuid\":\"c874527c-990c-4788-aa16-7f8a0c94d194\"},{\"content\":{\"side\":\"TOP\"},\"type\":\"ConnectorPlacement.EquallySpacedRectSide\",\"uuid\":\"b0161d26-106e-466a-8756-17981005591c\"},{\"content\":{\"connectorIds\":[\"In2\",\"In3\"],\"side\":\"BOTTOM\"},\"type\":\"ConnectorPlacement.EquallySpacedRectSide\",\"uuid\":\"87eba4bb-8cc6-4d91-843e-d033b71d377b\"}]},\"type\":\"ConnectorPlacement.EquallySpacedConnector\",\"uuid\":\"031ea5bd-d22b-4033-942a-a77822380b2b\"}],\"packageUris\":[\"http://schema.mathworks.com/mf0/Connector/R2020b\"],\"version\":\"1.0\"}"
  Filtre HF : eeGeneralControl/Low-Pass Filter (Discrete or Continuous)  K=1  T=0.00004  B=inf  A=-inf  init_option=Inherited from block input  x0=0  Ts=-1
  Filtre HF1 : eeGeneralControl/Low-Pass Filter (Discrete or Continuous)  K=1  T=0.00004  B=inf  A=-inf  init_option=Inherited from block input  x0=0  Ts=-1
  Mux1 : Mux  Inputs=2
  Mux2 : Mux  Inputs=2
  PID Controller1 : slpidlib/PID Controller  Controller=PI  Form=Parallel  TimeDomain=Continuous-time  UseExternalTs=off  SampleTime=Ts  IntegratorMethod=Forward Euler  FilterMethod=Forward Euler  ControllerParametersSource=internal  P=kp_isd  I=ki_isd  UseKiTs=off  D=0  UseExternalDerivativeSource=off  N=100  UseFilter=on  TunerSelectOption=Transfer Function Based (PID Tuner App)  InitialConditionSource=internal  InitialConditionForIntegrator=0  InitialConditionForFilter=0  DifferentiatorICPrevScaledInput=0  ExternalReset=none  TrackingMode=off  Kt=1  LimitOutput=off  SatLimitsSource=internal  UpperSaturationLimit=inf  LowerSaturationLimit=-inf  LinearizeAsGain=on  AntiWindupMode=none  Kb=1  LimitIntegrator=off  UpperIntegratorSaturationLimit=inf  LowerIntegratorSaturationLimit=-inf  POutMin=[]  POutMax=[]  IOutMin=[]  IOutMax=[]  DOutMin=[]  DOutMax=[]  NOutMin=[]  NOutMax=[]  SumOutMin=[]  SumOutMax=[]  SaturationOutMin=[]  SaturationOutMax=[]  PParamMin=[]  PParamMax=[]  IParamMin=[]  IParamMax=[]  DParamMin=[]  DParamMax=[]  NParamMin=[]  NParamMax=[]  KbParamMin=[]  KbParamMax=[]  KtParamMin=[]  KtParamMax=[]  KbOutMin=[]  KbOutMax=[]  KtOutMin=[]  KtOutMax=[]  IntegratorOutMin=[]  IntegratorOutMax=[]  FilterOutMin=[]  FilterOutMax=[]  SumI1OutMin=[]  SumI1OutMax=[]  SumI2OutMin=[]  SumI2OutMax=[]  SumI3OutMin=[]  SumI3OutMax=[]  SumI4OutMin=[]  SumI4OutMax=[]  SumDOutMin=[]  SumDOutMax=[]  DifferentiatorOutMin=[]  DifferentiatorOutMax=[]  FilterDiffOutCoefMin=[]  FilterDiffOutCoefMax=[]  ReciprocalOutMin=[]  ReciprocalOutMax=[]  SumDenOutMin=[]  SumDenOutMax=[]  SumNumOutMin=[]  SumNumOutMax=[]  DivideOutMin=[]  DivideOutMax=[]  UdiffTsProdOutMin=[]  UdiffTsProdOutMax=[]  NTsProdOutMin=[]  NTsProdOutMax=[]  UintegralTsProdOutMin=[]  UintegralTsProdOutMax=[]  UngainTsProdOutMin=[]  UngainTsProdOutMax=[]  ClampingZeroOutDataTypeStr=Inherit: Inherit via back propagation  ClampingZeroOutMin=[]  ClampingZeroOutMax=[]  FilterDenConstantOutDataTypeStr=Inherit: Inherit via back propagation  FilterDenConstantOutMin=[]  FilterDenConstantOutMax=[]  PCopyOutDataTypeStr=Inherit: Inherit via back propagation  PCopyOutMin=[]  PCopyOutMax=[]  NCopyOutDataTypeStr=Inherit: Inherit via back propagation  NCopyOutMin=[]  NCopyOutMax=[]  IntegratorContinuousStateAttributes=''  IntegratorStateMustResolveToSignalObject=off  IntegratorRTWStateStorageClass=Auto  FilterContinuousStateAttributes=''  FilterStateMustResolveToSignalObject=off  FilterRTWStateStorageClass=Auto  ParallelPVariant=InternalParameters  IdealPVariant=Disabled  IVariant=InternalParameters  DVariant=Disabled  IntegratorVariant=Continuous  SatVariant=Disabled  AWVariant=Passthrough  PCopyVariant=Disabled  TRVariant=Disabled  FdbkBlocksVariant=Forward  IdealPFdbkVariant=Disabled  SatFdbkVariant=Disabled  DerivativeFilterVariant=Disabled  NVariant=Disabled  NCopyVariant=Disabled_SignalSpec  FilterICVariant=Disabled  IntegratorICVariant=InternalICs  ExternalResetVariant=Disabled  TRSumVariant=Passthrough  SumFdbkVariant=Disabled  SumVariant=Sum_PI  TsampFilterVariant=InternalTs  TsampNgainVariant=Passthrough  TsampIntegralVariant=Disabled_SignalSpec  ExternalSaturationOutDataTypeStr=Inherit: Same as second input  DerivativeSourceVariant=Disabled
  Sum : Sum  Inputs=+-
  boucle isd : Scope
  Vdref : Outport
  tag scope: isd_ref=global, vd=global
  wires:
  Id/1 -> Mux1/1, Sum/2
  [I_sq] -> Filtre HF/1
  [Omega_G] -> Découplage Axe d/3(Wm)
  Mux1/1 -> boucle isd/1
  Id_ref/1 -> Sum/1, Mux1/2, [isd_ref]
  Sum/1 -> PID Controller1/1
  Découplage Axe d/1(Vdref) -> Mux2/2, Vdref/1
  PID Controller1/1 -> Filtre HF1/1, Découplage Axe d/1(vd), Mux2/1, [vd]
  Filtre HF/1 -> Découplage Axe d/2(Iq)
  Mux2/1 -> " Vd/Vdref"/1

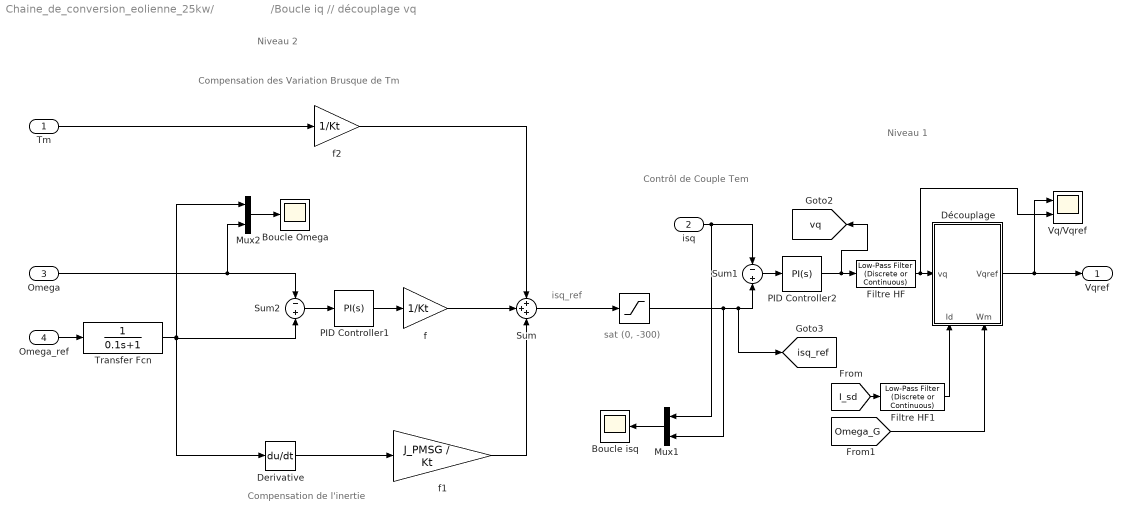
== system Chaine_de_conversion_eolienne_25kw/                 /Boucle iq // découplage vq ==
  note: sat (0, -300)
  note: Compensation des Variation Brusque de Tm
  note: isq_ref
  note: Compensation de l'inertie
  note: Contrôl de Couple Tem
  note: Niveau 1
  note: Niveau 2
  Tm : Inport
  isq : Inport  Port=2
  Omega : Inport  Port=3
  Omega_ref : Inport  Port=4
  "  " : Saturate  UpperLimit=0  LowerLimit=-300
  "Boucle Omega " : Scope
  Boucle isq : Scope
  Derivative : Derivative
  Découplage : Subsystem
      settings: PortSchema="{\"entries\":[{\"content\":{\"sides\":[{\"content\":{\"connectorIds\":[\"In1\"]},\"type\":\"ConnectorPlacement.EquallySpacedRectSide\",\"uuid\":\"a35b541f-6c91-4579-89f1-6689e9beed7f\"},{\"content\":{\"connectorIds\":[\"Out1\"],\"side\":\"RIGHT\"},\"type\":\"ConnectorPlacement.EquallySpacedRectSide\",\"uuid\":\"c874527c-990c-4788-aa16-7f8a0c94d194\"},{\"content\":{\"side\":\"TOP\"},\"type\":\"ConnectorPlacement.EquallySpacedRectSide\",\"uuid\":\"b0161d26-106e-466a-8756-17981005591c\"},{\"content\":{\"connectorIds\":[\"In2\",\"In3\"],\"side\":\"BOTTOM\"},\"type\":\"ConnectorPlacement.EquallySpacedRectSide\",\"uuid\":\"6bea0741-ba37-48dd-9c1f-2166530afd2a\"}]},\"type\":\"ConnectorPlacement.EquallySpacedConnector\",\"uuid\":\"031ea5bd-d22b-4033-942a-a77822380b2b\"}],\"packageUris\":[\"http://schema.mathworks.com/mf0/Connector/R2020b\"],\"version\":\"1.0\"}"
  Filtre HF : eeGeneralControl/Low-Pass Filter (Discrete or Continuous)  K=1  T=0.00004  B=inf  A=-inf  init_option=Inherited from block input  x0=0  Ts=-1
  Filtre HF1 : eeGeneralControl/Low-Pass Filter (Discrete or Continuous)  K=1  T=0.00004  B=inf  A=-inf  init_option=Inherited from block input  x0=0  Ts=-1
  Mux1 : Mux  Inputs=2
  Mux2 : Mux  Inputs=2
  PID Controller1 : slpidlib/PID Controller  Controller=PI  Form=Parallel  TimeDomain=Continuous-time  UseExternalTs=off  SampleTime=Ts  IntegratorMethod=Forward Euler  FilterMethod=Forward Euler  ControllerParametersSource=internal  P=kp_omega  I=ki_omega  UseKiTs=off  D=0  UseExternalDerivativeSource=off  N=100  UseFilter=on  TunerSelectOption=Transfer Function Based (PID Tuner App)  InitialConditionSource=internal  InitialConditionForIntegrator=0  InitialConditionForFilter=0  DifferentiatorICPrevScaledInput=0  ExternalReset=none  TrackingMode=off  Kt=1  LimitOutput=off  SatLimitsSource=internal  UpperSaturationLimit=222.3  LowerSaturationLimit=0  LinearizeAsGain=on  AntiWindupMode=back-calculation  Kb=1  LimitIntegrator=off  UpperIntegratorSaturationLimit=inf  LowerIntegratorSaturationLimit=-inf  POutMin=[]  POutMax=[]  IOutMin=[]  IOutMax=[]  DOutMin=[]  DOutMax=[]  NOutMin=[]  NOutMax=[]  SumOutMin=[]  SumOutMax=[]  SaturationOutMin=[]  SaturationOutMax=[]  PParamMin=[]  PParamMax=[]  IParamMin=[]  IParamMax=[]  DParamMin=[]  DParamMax=[]  NParamMin=[]  NParamMax=[]  KbParamMin=[]  KbParamMax=[]  KtParamMin=[]  KtParamMax=[]  KbOutMin=[]  KbOutMax=[]  KtOutMin=[]  KtOutMax=[]  IntegratorOutMin=[]  IntegratorOutMax=[]  FilterOutMin=[]  FilterOutMax=[]  SumI1OutMin=[]  SumI1OutMax=[]  SumI2OutMin=[]  SumI2OutMax=[]  SumI3OutMin=[]  SumI3OutMax=[]  SumI4OutMin=[]  SumI4OutMax=[]  SumDOutMin=[]  SumDOutMax=[]  DifferentiatorOutMin=[]  DifferentiatorOutMax=[]  FilterDiffOutCoefMin=[]  FilterDiffOutCoefMax=[]  ReciprocalOutMin=[]  ReciprocalOutMax=[]  SumDenOutMin=[]  SumDenOutMax=[]  SumNumOutMin=[]  SumNumOutMax=[]  DivideOutMin=[]  DivideOutMax=[]  UdiffTsProdOutMin=[]  UdiffTsProdOutMax=[]  NTsProdOutMin=[]  NTsProdOutMax=[]  UintegralTsProdOutMin=[]  UintegralTsProdOutMax=[]  UngainTsProdOutMin=[]  UngainTsProdOutMax=[]  ClampingZeroOutDataTypeStr=Inherit: Inherit via back propagation  ClampingZeroOutMin=[]  ClampingZeroOutMax=[]  FilterDenConstantOutDataTypeStr=Inherit: Inherit via back propagation  FilterDenConstantOutMin=[]  FilterDenConstantOutMax=[]  PCopyOutDataTypeStr=Inherit: Inherit via back propagation  PCopyOutMin=[]  PCopyOutMax=[]  NCopyOutDataTypeStr=Inherit: Inherit via back propagation  NCopyOutMin=[]  NCopyOutMax=[]  IntegratorContinuousStateAttributes=''  IntegratorStateMustResolveToSignalObject=off  IntegratorRTWStateStorageClass=Auto  FilterContinuousStateAttributes=''  FilterStateMustResolveToSignalObject=off  FilterRTWStateStorageClass=Auto  ParallelPVariant=InternalParameters  IdealPVariant=Disabled  IVariant=InternalParameters  DVariant=Disabled  IntegratorVariant=Continuous  SatVariant=Disabled  AWVariant=Passthrough  PCopyVariant=Disabled  TRVariant=Disabled  FdbkBlocksVariant=Forward  IdealPFdbkVariant=Disabled  SatFdbkVariant=Disabled  DerivativeFilterVariant=Disabled  NVariant=Disabled  NCopyVariant=Disabled_SignalSpec  FilterICVariant=Disabled  IntegratorICVariant=InternalICs  ExternalResetVariant=Disabled  TRSumVariant=Passthrough  SumFdbkVariant=Disabled  SumVariant=Sum_PI  TsampFilterVariant=InternalTs  TsampNgainVariant=Passthrough  TsampIntegralVariant=Disabled_SignalSpec  ExternalSaturationOutDataTypeStr=Inherit: Same as second input  DerivativeSourceVariant=Disabled
  PID Controller2 : slpidlib/PID Controller  Controller=PI  Form=Parallel  TimeDomain=Continuous-time  UseExternalTs=off  SampleTime=Ts  IntegratorMethod=Forward Euler  FilterMethod=Forward Euler  ControllerParametersSource=internal  P=kp_isd  I=ki_isd  UseKiTs=off  D=0  UseExternalDerivativeSource=off  N=100  UseFilter=on  TunerSelectOption=Transfer Function Based (PID Tuner App)  InitialConditionSource=internal  InitialConditionForIntegrator=0  InitialConditionForFilter=0  DifferentiatorICPrevScaledInput=0  ExternalReset=none  TrackingMode=off  Kt=1  LimitOutput=off  SatLimitsSource=internal  UpperSaturationLimit=inf  LowerSaturationLimit=-inf  LinearizeAsGain=on  AntiWindupMode=none  Kb=1  LimitIntegrator=off  UpperIntegratorSaturationLimit=inf  LowerIntegratorSaturationLimit=-inf  POutMin=[]  POutMax=[]  IOutMin=[]  IOutMax=[]  DOutMin=[]  DOutMax=[]  NOutMin=[]  NOutMax=[]  SumOutMin=[]  SumOutMax=[]  SaturationOutMin=[]  SaturationOutMax=[]  PParamMin=[]  PParamMax=[]  IParamMin=[]  IParamMax=[]  DParamMin=[]  DParamMax=[]  NParamMin=[]  NParamMax=[]  KbParamMin=[]  KbParamMax=[]  KtParamMin=[]  KtParamMax=[]  KbOutMin=[]  KbOutMax=[]  KtOutMin=[]  KtOutMax=[]  IntegratorOutMin=[]  IntegratorOutMax=[]  FilterOutMin=[]  FilterOutMax=[]  SumI1OutMin=[]  SumI1OutMax=[]  SumI2OutMin=[]  SumI2OutMax=[]  SumI3OutMin=[]  SumI3OutMax=[]  SumI4OutMin=[]  SumI4OutMax=[]  SumDOutMin=[]  SumDOutMax=[]  DifferentiatorOutMin=[]  DifferentiatorOutMax=[]  FilterDiffOutCoefMin=[]  FilterDiffOutCoefMax=[]  ReciprocalOutMin=[]  ReciprocalOutMax=[]  SumDenOutMin=[]  SumDenOutMax=[]  SumNumOutMin=[]  SumNumOutMax=[]  DivideOutMin=[]  DivideOutMax=[]  UdiffTsProdOutMin=[]  UdiffTsProdOutMax=[]  NTsProdOutMin=[]  NTsProdOutMax=[]  UintegralTsProdOutMin=[]  UintegralTsProdOutMax=[]  UngainTsProdOutMin=[]  UngainTsProdOutMax=[]  ClampingZeroOutDataTypeStr=Inherit: Inherit via back propagation  ClampingZeroOutMin=[]  ClampingZeroOutMax=[]  FilterDenConstantOutDataTypeStr=Inherit: Inherit via back propagation  FilterDenConstantOutMin=[]  FilterDenConstantOutMax=[]  PCopyOutDataTypeStr=Inherit: Inherit via back propagation  PCopyOutMin=[]  PCopyOutMax=[]  NCopyOutDataTypeStr=Inherit: Inherit via back propagation  NCopyOutMin=[]  NCopyOutMax=[]  IntegratorContinuousStateAttributes=''  IntegratorStateMustResolveToSignalObject=off  IntegratorRTWStateStorageClass=Auto  FilterContinuousStateAttributes=''  FilterStateMustResolveToSignalObject=off  FilterRTWStateStorageClass=Auto  ParallelPVariant=InternalParameters  IdealPVariant=Disabled  IVariant=InternalParameters  DVariant=Disabled  IntegratorVariant=Continuous  SatVariant=Disabled  AWVariant=Passthrough  PCopyVariant=Disabled  TRVariant=Disabled  FdbkBlocksVariant=Forward  IdealPFdbkVariant=Disabled  SatFdbkVariant=Disabled  DerivativeFilterVariant=Disabled  NVariant=Disabled  NCopyVariant=Disabled_SignalSpec  FilterICVariant=Disabled  IntegratorICVariant=InternalICs  ExternalResetVariant=Disabled  TRSumVariant=Passthrough  SumFdbkVariant=Disabled  SumVariant=Sum_PI  TsampFilterVariant=InternalTs  TsampNgainVariant=Passthrough  TsampIntegralVariant=Disabled_SignalSpec  ExternalSaturationOutDataTypeStr=Inherit: Same as second input  DerivativeSourceVariant=Disabled
  Sum : Sum  Inputs=+++
  Sum1 : Sum  Inputs=-+
  Sum2 : Sum  Inputs=-+
  Transfer Fcn : TransferFcn  Denominator=[0.1 1]
  Vq/Vqref : Scope  NumInputPorts=2
  f : Gain  Gain=1/Kt  SaturateOnIntegerOverflow=on  OutDataTypeStr=Inherit: Same as input  ParamDataTypeStr=Inherit: Same as input
  f1 : Gain  Gain=J_PMSG / Kt  SaturateOnIntegerOverflow=on  OutDataTypeStr=Inherit: Same as input  ParamDataTypeStr=Inherit: Same as input
  f2 : Gain  Gain=1/Kt  SaturateOnIntegerOverflow=on  OutDataTypeStr=Inherit: Same as input  ParamDataTypeStr=Inherit: Same as input
  Vqref : Outport
  tag scope: isq_ref=global, vq=global
  wires:
  [I_sd] -> Filtre HF1/1
  Mux1/1 -> Boucle isq/1
  Omega/1 -> Mux2/2, Sum2/1
  isq/1 -> Sum1/1, Mux1/1
  PID Controller2/1 -> [vq], Filtre HF/1
  Sum1/1 -> PID Controller2/1
  Sum2/1 -> PID Controller1/1
  Mux2/1 -> "Boucle Omega "/1
  PID Controller1/1 -> f/1
  Tm/1 -> f2/1
  Derivative/1 -> f1/1
  Découplage/1(Vqref) -> Vqref/1, Vq/Vqref/1
  Filtre HF/1 -> Vq/Vqref/2, Découplage/1(vq)
  Filtre HF1/1 -> Découplage/2(Id)
  [Omega_G] -> Découplage/3(Wm)
  "  "/1 -> Mux1/2, [isq_ref], Sum1/2
  f/1 -> Sum/2
  Sum/1 -> "  "/1
  f2/1 -> Sum/1
  Transfer Fcn/1 -> Derivative/1, Sum2/2, Mux2/1
  Omega_ref/1 -> Transfer Fcn/1
  f1/1 -> Sum/3

== system Chaine_de_conversion_eolienne_25kw/                 /Générateur  PWM ==
  abc_ref : Inport
  Divide3 : Product  Inputs=*/
  PWM Generator (2-Level) : spsPWMGenerator2LevelLib/PWM Generator (2-Level)  ModulatorType=Three-phase bridge (6 pulses)  ModulatorMode=Unsynchronized  Fc=Fc  Pc=90  nF=27  MinMax="[ -1  1 ]"  SamplingTechnique=Natural  ModulatingSignals=off  m=0.8  Freq=60  Phase=0  Ts=Ts  ShowCarrierOutport=off
  Scope : Scope
  Unit Delay1 : UnitDelay  SampleTime=Ts  HasFrameUpgradeWarning=on
  indiceM=33_(1/(fr*33)3 : Constant  Value=Vdc_ref/2
  Commandes de Redresseur : Outport
  wires:
  indiceM=33_(1/(fr*33)3/1 -> Divide3/2
  abc_ref/1 -> Divide3/1
  PWM Generator (2-Level)/1 -> Commandes de Redresseur/1
  Unit Delay1/1 -> PWM Generator (2-Level)/1, Scope/1
  Divide3/1 -> Unit Delay1/1
